simulink model "vx_vy_dekf_v1_12"  (R2024a)
settings: Solver=VariableStepAuto  StartTime=0.0  StopTime=16  RelTol=1e-3
model workspace (MAT data in the model file):
  AVz_bias_v17 = 0
  Ay_bias_v17 = 0
  Q_r_v16 = 0.001
  Q_vy_v16 = 0.0001
  R_Ay_v14 = 0.01
  R_Ay_v15 = 0.01
  R_r_v14 = 0.01
  R_r_v15 = 0.01
  test_speed = 20
  test_steer_amplitude = 0.02
  test_steer_frequency = 0.4
undefined symbols (not defined in the file or in its folder): longitudinal_velocity_estimator_simulink, vy_dekf_v1_12_steer_profile, vy_dynamic_ekf_v1_7
libraries: simulink x4, Solver_SF x1
settings Model: Creator=Xiao Hu  LastModifiedBy=21180

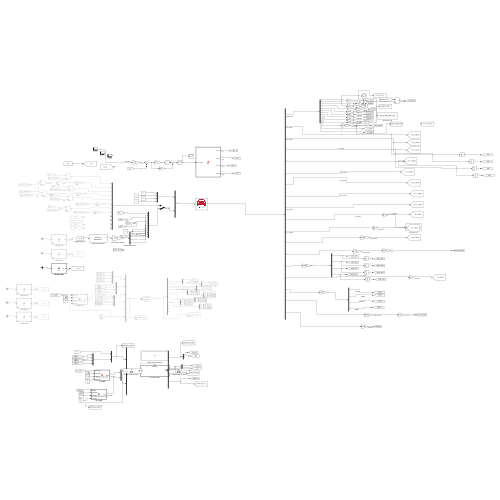
[thumbnail: Simulink's stored preview of the top-level diagram]
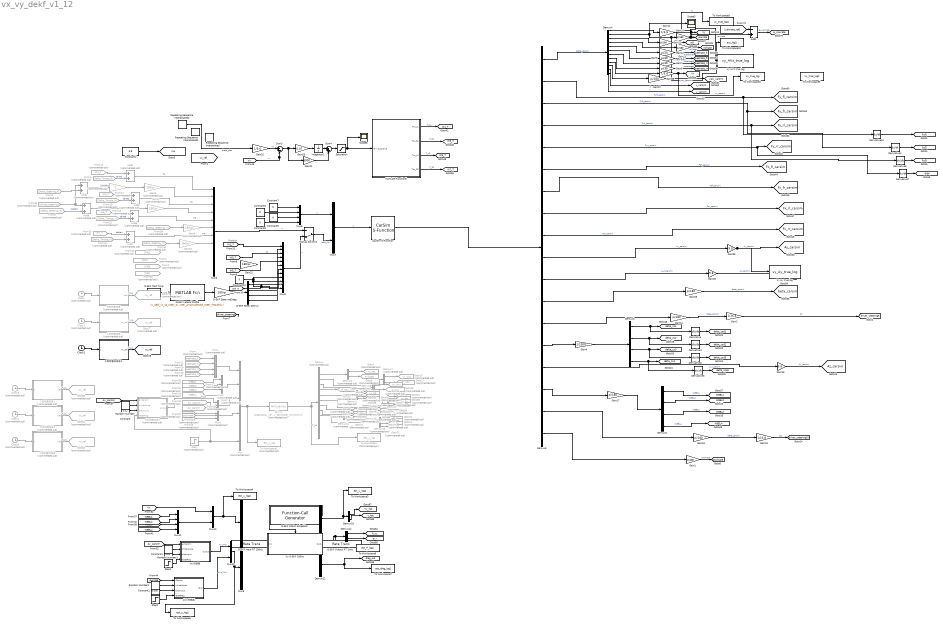
== system vx_vy_dekf_v1_12 ==
  note: Product
  AVz传感器 : MATLAB Function  TreatAsAtomicUnit=on  SystemSampleTime=0.01
  Add1 : Sum  Inputs=-+
  Add{4..9} (6 alike) : Sum  Commented=on
  B高附着加速 : MATLAB Function  Commented=on  TreatAsAtomicUnit=on
  CarSim S-Function : Solver_SF/CarSim S-Function  Priority=1  SIMFILE=simfile.sim  Run_RTs=off  vs_state_ind=Run  StopMode_ind=Vehicle Model
  Clock{,1,3..5} (5 alike) : Clock  Commented=on
  Clock2 : Clock
  Constant : Constant  Value=0.02
  Constant1 : Constant  Value=0.02
  Constant{6..10} (5 alike) : Constant  Value=0
  Constant2 : Constant  Value=0.005
  Constant4 : Constant  Value=0.8
  C高附着减速 : MATLAB Function  Commented=on  TreatAsAtomicUnit=on
  D-EKF 100Hz Scheduler : simulink/Ports & Subsystems/Function-Call Generator  sample_time=0.01  numberOfIterations=1  DisallowWideOutput=off
  D-EKF Input RT 100Hz : RateTransition  OutPortSampleTime=0.01
  D-EKF Lateral Profile : MATLABFcn  MATLABFcn=vy_dekf_v1_12_steer_profile(u,test_steer_amplitude,test_steer_frequency)  OutputDimensions=4  SampleTime=0.001
  D-EKF Output RT 1kHz : RateTransition  OutPortSampleTime=0.001
  D-EKF Steer Demux : Demux
  D-EKF Steer rad2deg : Gain  Gain=180/pi
  D-EKF Test Time : DigitalClock  SampleTime=0.001
  Demux : Demux  Commented=on  Outputs=[2 2 2 1 4 4 4 4 4 2 2 7]
  Demux{1,9..11,13} (5 alike) : Demux  Commented=on
  Demux12 : Demux  Outputs=[2 2 47]
  Demux14 : Demux  Outputs=2
  Demux18 : Demux  Outputs=2
  Demux2 : Demux  Commented=on  Outputs=2
  Demux3 : Demux
  Demux4 : Demux  Outputs=12
  Demux5 : Demux  Outputs=[12 1 1 1 1 1 1 1 1 1 1 1 1 4 1 4 1 1]
  Demux6 : Demux
  Demux7 : Demux  Commented=on  Outputs=2
  Demux8 : Demux  Commented=on  Outputs=2
  Derivative{,1..4,6..7,12} (8 alike) : Derivative
  D高附着加减速1 : MATLAB Function  TreatAsAtomicUnit=on
  From : From  Commented=on  GotoTag=weelrate_fl  TagVisibility=global
  From11 : From  Commented=on  GotoTag=weelrate_fr  TagVisibility=global
  From12 : From  Commented=on  GotoTag=W5_T  TagVisibility=global
  From13 : From  Commented=on  GotoTag=W1_T  TagVisibility=global
  From14 : From  Commented=on  GotoTag=weelrate_rl  TagVisibility=global
  From15 : From  Commented=on  GotoTag=weelrate_rr  TagVisibility=global
  From16 : From  Commented=on  GotoTag=WEEL1  TagVisibility=global
  From17 : From  Commented=on  GotoTag=WEEL3  TagVisibility=global
  From18 : From  Commented=on  GotoTag=WEEL2  TagVisibility=global
  From19 : From  Commented=on  GotoTag=WEEL4  TagVisibility=global
  From2 : From  Commented=on  GotoTag=Fd2  TagVisibility=global
  From20 : From  Commented=on  GotoTag=yawrate  TagVisibility=global
  From21 : From  Commented=on  GotoTag=W3_T  TagVisibility=global
  From22 : From  Commented=on  GotoTag=Delta_Torque_rl  TagVisibility=global
  From23 : From  Commented=on  GotoTag=Delta_Torque_fr  TagVisibility=global
  From24 : From  Commented=on  GotoTag=Delta_Torque_rr  TagVisibility=global
  From25 : From  Commented=on  GotoTag=rollrate  TagVisibility=global
  From26 : From  Commented=on  GotoTag=Ay_carsim  TagVisibility=global
  From28 : From  Commented=on  GotoTag=Az_carsim  TagVisibility=global
  From29 : From  Commented=on  GotoTag=W7_T  TagVisibility=global
  From3 : From  Commented=on  GotoTag=Delta_Torque_fl  TagVisibility=global
  From30 : From  Commented=on  GotoTag=pitchrate  TagVisibility=global
  From35 : From  Commented=on  GotoTag=driver_steering
  From39 : From  Commented=on  GotoTag=Delta_Steering_rl  TagVisibility=global
  From4 : From  Commented=on  GotoTag=Fd3  TagVisibility=global
  From42 : From  Commented=on  GotoTag=Delta_Steering_rr  TagVisibility=global
  From43 : From  Commented=on  GotoTag=Fd1  TagVisibility=global
  From5 : From  Commented=on  GotoTag=Delta_Steering_fl  TagVisibility=global
  From50 : From  Commented=on  GotoTag=Fd4  TagVisibility=global
  From6 : From  Commented=on  GotoTag=Delta_Steering_fr  TagVisibility=global
  F低附着加速1 : MATLAB Function  Commented=on  TreatAsAtomicUnit=on
  F低附着加速2 : MATLAB Function  Commented=on  TreatAsAtomicUnit=on
  Gain{1,10,12,14,17..18,23,29,37} (9 alike) : Gain  Gain=pi/180
  Gain11 : Gain  Gain=1/3.6
  Gain{3,5,9,13} (4 alike) : Gain  Commented=on  Gain=180/pi
  Gain15 : Gain  Gain=1/3.6
  Gain16 : Gain  Gain=9.8
  Gain19 : Gain  Gain=1/16.8
  Gain2 : Gain  Gain=1/16.8
  Gain21 : Gain  Gain=5000
  Gain22 : Gain  Gain=180/pi
  Gain{6..8,24} (4 alike) : Gain  Gain=pi/30
  Gain25 : Gain  Gain=0.07
  Gain28 : Gain  Gain=9.8
  Gain36 : Gain  Gain=9.8
  Gain38 : Gain  Gain=1/3.6
  Gain39 : Gain  Commented=on
  Gain4 : Gain  Gain=1/1000
  Goto10 : Goto  Commented=on  GotoTag=vx_wss  TagVisibility=global
  Goto17 : Goto  Commented=on  GotoTag=P_wss  TagVisibility=global
  Goto28 : Goto  Commented=on  GotoTag=vx_imu  TagVisibility=global
  Goto29 : Goto  Commented=on  GotoTag=P_imu  TagVisibility=global
  Goto30 : Goto  Commented=on  GotoTag=P_wss_imu  TagVisibility=global
  Goto32 : Goto  Commented=on  GotoTag=vx_FL  TagVisibility=global
  Goto38 : Goto  Commented=on  GotoTag=vx_FR  TagVisibility=global
  Goto39 : Goto  Commented=on  GotoTag=vx_RL  TagVisibility=global
  Goto40 : Goto  Commented=on  GotoTag=vx_RR  TagVisibility=global
  Goto41 : Goto  Commented=on  GotoTag=slip_FL  TagVisibility=global
  Goto57 : Goto  Commented=on  GotoTag=slip_FR  TagVisibility=global
  Goto58 : Goto  Commented=on  GotoTag=slip_RL  TagVisibility=global
  Goto59 : Goto  Commented=on  GotoTag=slip_RR  TagVisibility=global
  Goto64 : Goto  Commented=on  GotoTag=rho_FL  TagVisibility=global
  Goto65 : Goto  Commented=on  GotoTag=rho_FR  TagVisibility=global
  Goto66 : Goto  Commented=on  GotoTag=rho_RL  TagVisibility=global
  Goto67 : Goto  Commented=on  GotoTag=rho_RR  TagVisibility=global
  Goto68 : Goto  Commented=on  GotoTag=R_FL  TagVisibility=global
  Goto69 : Goto  Commented=on  GotoTag=R_FR  TagVisibility=global
  Goto7 : Goto  Commented=on  GotoTag=vx_hat  TagVisibility=global
  Goto70 : Goto  Commented=on  GotoTag=R_RL  TagVisibility=global
  Goto71 : Goto  Commented=on  GotoTag=R_RR  TagVisibility=global
  Goto72 : Goto  Commented=on  GotoTag=R_FL  TagVisibility=global
  Goto73 : Goto  Commented=on  GotoTag=R_FR  TagVisibility=global
  Goto74 : Goto  Commented=on  GotoTag=R_RL  TagVisibility=global
  Goto75 : Goto  Commented=on  GotoTag=R_RR  TagVisibility=global
  Goto{76..77,80..82} (5 alike) : Goto  Commented=on  GotoTag=vx_ref  TagVisibility=global
  Goto9 : Goto  Commented=on  GotoTag=P_fused  TagVisibility=global
  G低附着减速2 : MATLAB Function  Commented=on  TreatAsAtomicUnit=on
  H低附着加减速 : MATLAB Function  Commented=on  TreatAsAtomicUnit=on
  Integrator1 : Integrator
  MATLAB Function5 : MATLAB Function  TreatAsAtomicUnit=on
  Manual Switch1 : ManualSwitch  CurrentSetting=0
  Mux : Mux  Commented=on  Inputs=[4 4 3 3 3 1]
  Mux1 : Mux  Commented=on
  Mux10 : Mux  Inputs=[1 4]
  Mux11 : Mux
  Mux12 : Mux  Inputs=2
  Mux2 : Mux  Commented=on
  Mux3 : Mux  Commented=on  Inputs=3
  Mux4 : Mux  Commented=on  Inputs=3
  Mux5 : Mux  Inputs=12
  Mux6 : Mux
  Mux7 : Mux  Inputs=[4,12]
  Mux8 : Mux  Inputs=12
  Mux9 : Mux  Inputs=[5 2]
  Random Number : RandomNumber  Variance=0.000025  Seed=20260819  SampleTime=0.01
  Random Number1 : RandomNumber  Variance=0.000025  Seed=20260819  SampleTime=0.01
  Random Number2 : RandomNumber  Variance=0.000025  Seed=20260819  SampleTime=0.01
  Repeating Sequence Interpolated : simulink/Sources/Repeating Sequence Interpolated  OutValues=[40 40 40 40].'  TimeValues=[0 3 8 16].'  LookUpMeth=Interpolation-Use End Values  tsamp=0.001  OutMin=[]  OutMax=[]  OutDataTypeStr=double  OutputDataTypeScalingMode=double  OutDataType=fixdt(0,8)  OutScaling=2^-10
  Repeating Sequence Interpolated1 : simulink/Sources/Repeating Sequence Interpolated  OutValues=[60 60 60 60].'  TimeValues=[0 3 8 16].'  LookUpMeth=Interpolation-Use End Values  tsamp=0.001  OutMin=[]  OutMax=[]  OutDataTypeStr=double  OutputDataTypeScalingMode=double  OutDataType=fixdt(0,8)  OutScaling=2^-10
  Repeating Sequence Interpolated2 : simulink/Sources/Repeating Sequence Interpolated  OutValues=test_speed*3.6*ones(4,1)  TimeValues=[0 3 8 16].'  LookUpMeth=Interpolation-Use End Values  tsamp=0.001  OutMin=[]  OutMax=[]  OutDataTypeStr=double  OutputDataTypeScalingMode=double  OutDataType=fixdt(0,8)  OutScaling=2^-10
  Saturation : Saturate  UpperLimit=2250  LowerLimit=-2250
  Scope3 : Scope
  Scope8 : Scope
  Step : Step  Commented=on  Time=0.01  Before=1  After=0  SampleTime=0
  Step1 : Step  Time=0.01  Before=1  After=0  SampleTime=0
  Step2 : Step  Time=0.01  Before=1  After=0  SampleTime=0
  Sum3 : Sum  Inputs=|+-
  Sum4 : Sum  Inputs=|++
  To Workspace : ToWorkspace  Commented=on  VariableName=est_y_log  SaveFormat=Timeseries  SampleTime=-1
  To Workspace1 : ToWorkspace  Commented=on  VariableName=est_u_log  SaveFormat=Timeseries  SampleTime=-1
  To Workspace10 : ToWorkspace  VariableName=avz_log1  SaveFormat=Timeseries  SampleTime=-1
  To Workspace2 : ToWorkspace  VariableName=Vx_true_log  SaveFormat=Timeseries  SampleTime=-1
  To Workspace3 : ToWorkspace  VariableName=est_y_log1  SaveFormat=Timeseries  SampleTime=-1
  To Workspace4 : ToWorkspace  VariableName=est_u_log1  SaveFormat=Timeseries  SampleTime=-1
  To Workspace5 : ToWorkspace  VariableName=Vx_true_log2  SaveFormat=Timeseries  SampleTime=-1
  To Workspace6 : ToWorkspace  VariableName=est_z_log1  SaveFormat=Timeseries  SampleTime=-1
  To Workspace7 : ToWorkspace  VariableName=est_diag_log1  SaveFormat=Timeseries  SampleTime=-1
  To Workspace8 : ToWorkspace  VariableName=est_P_log1  SaveFormat=Timeseries  SampleTime=-1
  To Workspace9 : ToWorkspace  VariableName=vy_true_log1  SaveFormat=Timeseries  SampleTime=-1
  Vy AVz true log : ToWorkspace  VariableName=vy_AVz_true_log  SaveFormat=Timeseries  SampleTime=0.01
  Vy Ay true log : ToWorkspace  VariableName=vy_Ay_true_log  SaveFormat=Timeseries  SampleTime=0.01
  Vy D-EKF 100Hz : Subsystem  TreatAsAtomicUnit=on
  ay传感器 : MATLAB Function  TreatAsAtomicUnit=on  SystemSampleTime=0.01
  估计vx : MATLABFcn  Commented=on  MATLABFcn=longitudinal_velocity_estimator_simulink(u)  OutputDimensions=38
  tag scope: Ax_carsim=global, Ay_carsim=global, Az_carsim=global, Fx_fl_carsim=global, Fx_fr_carsim=global, Fx_rl_carsim=global, Fx_rr_carsim=global, Fy_fl_carsim=global, Fy_fr_carsim=global, Fy_rl_carsim=global, Fy_rr_carsim=global, P_r=global, P_vy=global, Vx=global, Vy=global, Vy_hat=global, W1_T=global, W3_T=global, W5_T=global, W7_T=global, WEEL1=global, WEEL2=global, WEEL3=global, WEEL4=global, beta_carsim=global, delta_zs1=global, delta_zs2=global, delta_zs3=global, delta_zs4=global, delta_zsd1=global, delta_zsd2=global, delta_zsd3=global, delta_zsd4=global, diag_out=global, driver_steering10=global, driver_steering5=global, e_yawrate=global, fyd1=global, fyd2=global, fyd3=global, fyd4=global, mu=global, pitchrate=global, r_hat=global, roll=global, rollrate=global, vx_ref=global, weelrate_fl=global, weelrate_fr=global, weelrate_rl=global, weelrate_rr=global, x_carsim=global, y_carsim=global, yaw_carsim=global, yawrate=global
  wires:
  From13/1 -> Add4/1
  Gain14/1 -> Gain2/1  "beta_carsim"
  Add1/1 -> [e_yawrate]  "e_yawrate"
  Gain3/1 -> Mux5/4
  From6/1 -> Add8/2  "delta3"
  [W1_T] -> Mux8/1
  Demux5/7 -> [Fx_fr_carsim]  "Fzfr_carsim"
  Demux3/4 -> Derivative3/1, [delta_zs4]
  From12/1 -> Add6/1
  From35/1 -> Add9/1, Add8/1
  Gain39/1 -> Gain5/1
  Gain13/1 -> Mux5/8
  Demux6/4 -> [WEEL4]  "WEEL4"
  Constant6/1 -> Mux6/2
  Add9/1 -> Gain39/1  "总的转角1"
  Derivative1/1 -> [delta_zsd2]
  Demux5/12 -> Gain29/1
  Demux5/8 -> [Fx_rl_carsim]  "Fzrl_carsim"
  Gain19/1 -> [driver_steering10]  "ds1"
  Add4/1 -> Mux5/1  "T1"
  Gain4/1 -> Demux3/1
  Gain38/1 -> To Workspace2/1, [Vx]  "vx_carsim"
  Gain8/1 -> [weelrate_rr]  "weelrate4"
  Add5/1 -> Mux5/3  "T2"
  Demux6/3 -> [WEEL2]  "WEEL2"
  Mux7/1 -> CarSim S-Function/1  "u"
  Mux8/1 -> Manual Switch1/2  "u"
  From21/1 -> Add5/1
  MATLAB Function5/2(Tor_R1) -> [W3_T]  "T_R1"
  Gain36/1 -> [Ay_carsim], Vy Ay true log/1  "Ay_carsim"
  Derivative3/1 -> [delta_zsd4]
  Gain11/1 -> To Workspace9/1, [Vy]  "Vy"
  Sum4/1 -> Saturation/1
  Gain9/1 -> Mux5/6
  Demux5/4 -> Derivative6/1, [Fy_rl_carsim]  "Fyrl_carsim"
  Gain5/1 -> Mux5/2
  Demux5/16 -> Gain17/1
  Gain21/1 -> Sum4/2
  CarSim S-Function/1 -> Demux5/1
  Derivative4/1 -> [fyd2]
  From39/1 -> Gain9/1
  From22/1 -> Add6/2  "delta3"
  Derivative12/1 -> [fyd1]
  From23/1 -> Add5/2  "delta2"
  Gain18/1 -> Gain19/1  "beta_carsim"
  Gain7/1 -> [weelrate_rl]  "weelrate3"
  Derivative7/1 -> [fyd4]
  Derivative6/1 -> [fyd3]
  Constant9/1 -> Mux6/3
  Mux6/1 -> Mux7/1  "u"
  [W3_T] -> Mux8/3  "q1"
  Gain12/1 -> [roll]  "roll"
  Gain17/1 -> Demux6/1
  Demux5/17 -> Gain18/1
  Demux6/2 -> [WEEL3]  "WEEL3"
  Gain16/1 -> [Az_carsim]  "Ax_carsim"
  Derivative/1 -> [delta_zsd1]
  Demux6/1 -> [WEEL1]  "WEEL1"
  Constant10/1 -> Mux8/12, Mux8/11, Mux8/10, Mux8/9
  MATLAB Function5/4(Tor_R2) -> [W7_T]  "T_R2"
  Demux5/13 -> Gain14/1
  Add6/1 -> Mux5/5  "T3"
  From5/1 -> Add9/2
  From3/1 -> Add4/2  "delta1"
  Demux4/7 -> Gain7/1
  MATLAB Function5/1(Tor_L1) -> [W1_T]  "T_L1"
  Demux3/3 -> Derivative2/1, [delta_zs3]
  Demux5/6 -> [Fx_fl_carsim]  "Fzfl_carsim"
  Constant4/1 -> [mu]
  Integrator1/1 -> Sum4/1
  Demux4/3 -> Gain12/1
  Demux5/5 -> [Fy_rr_carsim], Derivative7/1  "Fyrr_carsim"
  Demux4/6 -> Gain6/1
  Derivative2/1 -> [delta_zsd3]
  Gain2/1 -> [driver_steering5]  "ds"
  Demux4/11 -> [x_carsim]  "X"
  Constant8/1 -> Mux6/4
  Demux5/2 -> Derivative12/1, [Fy_fl_carsim]  "Fyfl_carsim"
  Gain6/1 -> [weelrate_fr]  "weelrate2"
  Demux5/1 -> Demux4/1  "delta_carsim"
  Demux5/11 -> Gain28/1  "w_rl_carsim"
  Demux4/5 -> Gain24/1
  Demux5/14 -> Gain4/1
  Add7/1 -> Mux5/7  "T4"
  Manual Switch1/1 -> Mux7/2  "add_Mz"
  Demux5/3 -> Derivative4/1, [Fy_fr_carsim]  "Fyfr_carsim"
  From24/1 -> Add7/2
  Demux4/12 -> [y_carsim]  "Y"
  Demux4/4 -> Gain23/1
  Demux4/2 -> Scope3/1, To Workspace10/1, Gain10/1
  Demux4/8 -> Gain8/1
  Demux5/10 -> Gain36/1  "Ay_carsim"
  Gain25/1 -> Integrator1/1
  Demux3/2 -> Derivative1/1, [delta_zs2]
  From29/1 -> Add7/1  "delta4"
  Gain37/1 -> [yaw_carsim]  "yaw_carsim"
  [driver_steering] -> ?
  Demux4/9 -> Gain38/1
  Demux3/1 -> Derivative/1, [delta_zs1]
  [W7_T] -> Mux8/7  "q1"
  [Vx] -> Sum3/2  "vx"
  Demux5/15 -> Gain16/1  "w_rl_carsim"
  Demux4/1 -> Gain11/1
  Gain28/1 -> [Ax_carsim]  "Ax_carsim"
  Gain24/1 -> [weelrate_fl]  "轮速实际值"
  From42/1 -> Gain13/1
  Constant7/1 -> Mux6/1
  Gain10/1 -> Add1/2, [yawrate], Vy AVz true log/1  "yawrate"
  [W5_T] -> Mux8/5
  Gain29/1 -> [beta_carsim]  "beta_carsim"
  Sum3/1 -> Gain25/1, Gain21/1
  Gain23/1 -> [rollrate]  "rollrate"
  MATLAB Function5/3(Tor_L2) -> [W5_T]  "T_L2"
  Mux5/1 -> Manual Switch1/1  "u"
  Add8/1 -> Gain3/1  "总的转角2"
  Demux4/10 -> Gain37/1
  Demux5/9 -> [Fx_rr_carsim]  "Fzrr_carsim"
  [yawrate_ref] -> Add1/1
  Mux/1 -> 估计vx/1, To Workspace1/1
  Mux1/1 -> Mux/1
  From/1 -> Mux1/1
  From11/1 -> Mux1/2
  From14/1 -> Mux1/3
  From15/1 -> Mux1/4
  From16/1 -> Mux2/1
  From17/1 -> Mux2/2
  From18/1 -> Mux2/3
  From19/1 -> Mux2/4
  Mux2/1 -> Mux/2
  Mux3/1 -> Mux/3
  Mux4/1 -> Mux/4
  Gain1/1 -> [pitchrate]  "pitchrate"
  Demux5/18 -> Gain1/1
  [Ax_carsim] -> F低附着加速2/1(axCarsim)
  From26/1 -> Mux3/2
  From28/1 -> Mux3/3
  From20/1 -> Mux4/1
  From30/1 -> Mux4/2
  From25/1 -> Mux4/3
  估计vx/1 -> Demux/1, To Workspace/1  "T_L1"
  Demux/1 -> Demux2/1
  Demux2/1 -> Goto7/1
  Demux2/2 -> Goto9/1
  Demux7/1 -> Goto10/1
  Demux/2 -> Demux7/1
  Demux7/2 -> Goto17/1
  Demux/3 -> Demux8/1
  Demux8/2 -> Goto29/1
  Demux8/1 -> Goto28/1
  Demux/4 -> Goto30/1
  Demux1/1 -> Goto32/1
  Demux1/2 -> Goto38/1
  Demux1/3 -> Goto39/1
  Demux1/4 -> Goto40/1
  Demux/5 -> Demux1/1
  Demux9/3 -> Goto58/1
  Demux/6 -> Demux9/1
  Demux9/4 -> Goto59/1
  Demux9/2 -> Goto57/1
  Demux9/1 -> Goto41/1
  Demux/7 -> Demux10/1
  Demux10/3 -> Goto66/1
  Demux10/1 -> Goto64/1
  Demux10/4 -> Goto67/1
  Demux10/2 -> Goto65/1
  Demux11/3 -> Goto70/1
  Demux11/4 -> Goto71/1
  Demux/8 -> Demux11/1
  Demux11/2 -> Goto69/1
  Demux11/1 -> Goto68/1
  Demux13/2 -> Goto73/1
  Demux/9 -> Demux13/1
  Demux13/3 -> Goto74/1
  Demux13/4 -> Goto75/1
  Demux13/1 -> Goto72/1
  Step/1 -> F低附着加速2/4(resetFlag), Mux/6
  Repeating Sequence Interpolated2/1 -> Gain15/1  "theta_des"
  Gain15/1 -> Sum3/1  "Vy"
  Clock/1 -> B高附着加速/1(t)
  B高附着加速/1(vref) -> Goto76/1  "T_L1"
  C高附着减速/1(Vx_ref) -> Goto77/1  "T_L1"
  Clock1/1 -> C高附着减速/1(t)
  Clock2/1 -> D高附着加减速1/1(t)
  D高附着加减速1/1(Vx_ref) -> [vx_ref]  "T_L1"
  Clock3/1 -> F低附着加速1/1(t)
  F低附着加速1/1(vref) -> Goto80/1  "T_L1"
  Saturation/1 -> Scope8/1, MATLAB Function5/1(Drive_torque)
  G低附着减速2/1(vref) -> Goto81/1  "T_L1"
  Clock4/1 -> G低附着减速2/1(t)
  H低附着加减速/1(vref) -> Goto82/1  "T_L1"
  Clock5/1 -> H低附着加减速/1(t)
  Constant/1 -> F低附着加速2/3(biasInput)
  Random Number/1 -> F低附着加速2/2(whiteNoise)
  F低附着加速2/1(axOut) -> Mux3/1  "T_L1"
  [Ay_carsim] -> ay传感器/1(ayCarsim)
  Demux18/2 -> [r_hat]
  Demux12/3 -> [diag_out], To Workspace7/1
  Demux12/1 -> To Workspace3/1, Demux18/1
  Step1/1 -> ay传感器/4(resetFlag)
  Constant1/1 -> ay传感器/3(biasInput)
  [WEEL3] -> Mux11/3
  [WEEL4] -> Mux11/4
  Random Number1/1 -> ay传感器/2(whiteNoise)
  [WEEL2] -> Mux11/2
  [WEEL1] -> Mux11/1
  Mux11/1 -> Mux10/2
  [Vx] -> Mux10/1
  Mux10/1 -> To Workspace4/1, Mux9/1
  ay传感器/1(ayOut) -> Mux12/1  "Ay_IMU"
  Mux12/1 -> Mux9/2, To Workspace6/1
  Random Number2/1 -> AVz传感器/2(whiteNoise)
  Constant2/1 -> AVz传感器/3(biasInput)
  Step2/1 -> AVz传感器/4(resetFlag)
  [yawrate] -> AVz传感器/1(rCarsim)
  AVz传感器/1(rOut) -> Mux12/2  "AVz_IMU"
  Demux18/1 -> [Vy_hat]
  Demux14/2 -> [P_r]
  Demux14/1 -> [P_vy]
  Demux12/2 -> To Workspace8/1, Demux14/1
  Mux9/1 -> D-EKF Input RT 100Hz/1
  D-EKF Input RT 100Hz/1 -> Vy D-EKF 100Hz/1(In1)
  D-EKF 100Hz Scheduler/1 -> Vy D-EKF 100Hz/Trigger
  Vy D-EKF 100Hz/1(Out1) -> D-EKF Output RT 1kHz/1
  D-EKF Output RT 1kHz/1 -> Demux12/1
  D-EKF Test Time/1 -> D-EKF Lateral Profile/1
  D-EKF Lateral Profile/1 -> D-EKF Steer rad2deg/1
  D-EKF Steer rad2deg/1 -> D-EKF Steer Demux/1
  D-EKF Steer Demux/1 -> Mux8/2
  D-EKF Steer Demux/2 -> Mux8/4
  D-EKF Steer Demux/3 -> Mux8/6
  D-EKF Steer Demux/4 -> Mux8/8

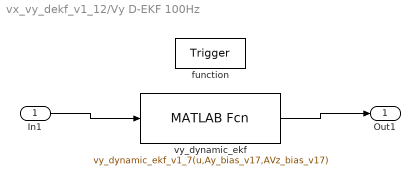
== system vx_vy_dekf_v1_12/Vy D-EKF 100Hz ==
  In1 : Inport
  function : TriggerPort  TriggerType=function-call  VariantControl=(inherit)
  vy_dynamic_ekf : MATLABFcn  MATLABFcn=vy_dynamic_ekf_v1_7(u,Ay_bias_v17,AVz_bias_v17)  OutputDimensions=51
  Out1 : Outport
  wires:
  In1/1 -> vy_dynamic_ekf/1
  vy_dynamic_ekf/1 -> Out1/1

== matlab function vx_vy_dekf_v1_12/B高附着加速 ==
  data: vref output; t input
function vref = fcn(t)

v0 = 60;
v1 = 100;

t1 = 3;
t2 = 8;

if t <= t1

    vref = v0;

elseif t < t2

    tau = (t-t1)/(t2-t1);

    s = 10*tau^3 ...
      - 15*tau^4 ...
      + 6*tau^5;

    vref = v0 + ...
        (v1-v0)*s;

else

    vref = v1;

end

== matlab function vx_vy_dekf_v1_12/C高附着减速 ==
  data: Vx_ref output; t input
function Vx_ref = fcn(t)
%#codegen
% 工况C：高附着直线平滑减速
% 0~3 s   : 100 km/h
% 3~8 s   : 100 -> 60 km/h
% 8~15 s  : 60 km/h
%
% 输出 Vx_ref 单位：m/s

v0 = 100;      % 27.7778 m/s
v1 = 60 ;       % 16.6667 m/s

t1 = 3.0;
t2 = 8.0;

if t <= t1

    Vx_ref = v0;

elseif t < t2

    tau = (t - t1) / (t2 - t1);

    s = 10*tau^3 - 15*tau^4 + 6*tau^5;

    Vx_ref = v0 + (v1 - v0)*s;

else

    Vx_ref = v1;

end
end

== matlab function vx_vy_dekf_v1_12/D高附着加减速1 ==
  data: Vx_ref output; t input
function Vx_ref = fcn(t)
%#codegen
% 加速-减速组合工况
%
% 0~3 s    : 60 km/h 匀速
% 3~8 s    : 60 -> 100 km/h 平滑加速
% 8~13 s   : 100 -> 60 km/h 平滑减速
% 13~16 s  : 60 km/h 匀速
%
% 输出 Vx_ref 单位：m/s

v_low  = 60;      % 16.6667 m/s
v_high = 100;
t1 = 3.0;
t2 = 8.0;
t3 = 13.0;

if t <= t1

    % 0~3 s：60 km/h 匀速
    Vx_ref = v_low;

elseif t < t2

    % 3~8 s：60 -> 100 km/h
    tau = (t - t1) / (t2 - t1);

    s = 10*tau^3 ...
      - 15*tau^4 ...
      + 6*tau^5;

    Vx_ref = v_low + (v_high - v_low)*s;

elseif t < t3

    % 8~13 s：100 -> 60 km/h
    tau = (t - t2) / (t3 - t2);

    s = 10*tau^3 ...
      - 15*tau^4 ...
      + 6*tau^5;

    Vx_ref = v_high + (v_low - v_high)*s;

else

    % 13~16 s：60 km/h 匀速
    Vx_ref = v_low;

end

end

== matlab function vx_vy_dekf_v1_12/F低附着加速1 ==
  data: vref output; t input
function vref = fcn(t)

% mu = 0.3
% 0~3 s : 40 km/h
% 3~8 s : 40 -> 70 km/h
% 8s以后: 70 km/h

v0 = 40;
v1 = 70;

t1 = 3;
t2 = 8;

if t <= t1

    vref_kmh = v0;

elseif t < t2

    tau = (t-t1)/(t2-t1);

    s = 10*tau^3 ...
      - 15*tau^4 ...
      + 6*tau^5;

    vref_kmh = v0 + ...
        (v1-v0)*s;

else

    vref_kmh = v1;

end

vref = vref_kmh;

end

== matlab function vx_vy_dekf_v1_12/G低附着减速2 ==
  data: vref output; t input
function vref = fcn(t)

% mu = 0.3
% 低附着平滑减速工况
%
% 0~3 s : 70 km/h
% 3~8 s : 70 -> 40 km/h
% 8s以后: 40 km/h
%
% 输出单位：km/h

v0 = 70;
v1 = 40;

t1 = 3;
t2 = 8;

if t <= t1

    vref_kmh = v0;

elseif t < t2

    tau = (t-t1)/(t2-t1);

    s = 10*tau^3 ...
      - 15*tau^4 ...
      + 6*tau^5;

    vref_kmh = v0 + ...
        (v1-v0)*s;

else

    vref_kmh = v1;

end

vref = vref_kmh;

end

== matlab function vx_vy_dekf_v1_12/H低附着加减速 ==
  data: vref output; t input
function vref = fcn(t)

% mu = 0.3
% 低附着加速-减速组合工况
%
% 0~3 s    : 40 km/h
% 3~8 s    : 40 -> 70 km/h
% 8~13 s   : 70 -> 40 km/h
% 13~16 s  : 40 km/h
%
% 输出单位：km/h

v_low  = 40;
v_high = 70;

t1 = 3;
t2 = 8;
t3 = 13;

if t <= t1

    % 0~3 s：40 km/h 匀速
    vref_kmh = v_low;

elseif t < t2

    % 3~8 s：40 -> 70 km/h 平滑加速
    tau = (t-t1)/(t2-t1);

    s = 10*tau^3 ...
      - 15*tau^4 ...
      + 6*tau^5;

    vref_kmh = v_low + ...
        (v_high-v_low)*s;

elseif t < t3

    % 8~13 s：70 -> 40 km/h 平滑减速
    tau = (t-t2)/(t3-t2);

    s = 10*tau^3 ...
      - 15*tau^4 ...
      + 6*tau^5;

    vref_kmh = v_high + ...
        (v_low-v_high)*s;

else

    % 13~16 s：40 km/h 匀速
    vref_kmh = v_low;

end

vref = vref_kmh;

end

== matlab function vx_vy_dekf_v1_12/F低附着加速2 ==
  data: axOut output; axCarsim input; whiteNoise input; biasInput input; resetFlag input
function axOut = imu_ax_preprocess( ...
    axCarsim, whiteNoise, biasInput, resetFlag)
%#codegen
%
% IMU纵向加速度传感器模型 + 因果低通预处理
%
% 输入：
%   axCarsim   : CarSim理想纵向加速度 [m/s^2]
%   whiteNoise : Random Number生成的白噪声 [m/s^2]
%   biasInput  : IMU残余bias [m/s^2]
%   resetFlag  : 与估计器reset一致
%
% 输出：
%   axOut      : 最终送入est_u(9)的IMU Ax
%
% 本模块按100Hz设计。

persistent yPrev

%% =========================================================
% 参数
% ==========================================================

Ts = 0.01;

% 第一版20 Hz低通
fc = 20.0;

%% =========================================================
% 输入数值保护
% ==========================================================

if ~isfinite(axCarsim)
    axCarsim = 0;
end

if ~isfinite(whiteNoise)
    whiteNoise = 0;
end

if ~isfinite(biasInput)
    biasInput = 0;
end

%% =========================================================
% 构造非理想IMU测量
%
% a_meas = a_true + bias + noise
% ==========================================================

axMeasured = ...
    axCarsim + ...
    biasInput + ...
    whiteNoise;

%% =========================================================
% 一阶因果低通参数
% ==========================================================

tau = ...
    1/(2*pi*fc);

alpha = ...
    Ts/(tau+Ts);

%% =========================================================
% 初始化 / reset
% ==========================================================

if isempty(yPrev)

    yPrev = axMeasured;

end

if resetFlag > 0.5

    yPrev = axMeasured;

end

%% =========================================================
% 因果一阶低通
%
% y[k] = y[k-1] + alpha*(x[k]-y[k-1])
% ==========================================================

axOut = ...
    yPrev + ...
    alpha*(axMeasured-yPrev);

%% =========================================================
% 保存
% ==========================================================

yPrev = axOut;

end

== matlab function vx_vy_dekf_v1_12/AVz传感器 ==
  data: rOut output; rCarsim input; whiteNoise input; biasInput input; resetFlag input
function rOut = imu_yawrate_preprocess( ...
    rCarsim, whiteNoise, biasInput, resetFlag)
%#codegen
%
% IMU横摆角速度传感器模型 + 一阶因果低通
%
% 输入：
%   rCarsim    : CarSim理想横摆角速度 AVz [rad/s]
%   whiteNoise : 陀螺仪白噪声 [rad/s]
%   biasInput  : 陀螺仪bias [rad/s]
%   resetFlag  : reset信号
%
% 输出：
%   rOut       : IMU处理后的横摆角速度 [rad/s]
%
% Sample time:
%   Ts = 0.01s
%   100Hz
%

persistent yPrev


%% ================================
% 参数
% ================================

Ts = 0.01;


% 陀螺仪低通截止频率
fc = 20;


%% ================================
% 初始化
% ================================

if isempty(yPrev)

    yPrev = 0;

end


%% ================================
% 数值保护
% ================================

if ~isfinite(rCarsim)

    rCarsim = 0;

end


if ~isfinite(whiteNoise)

    whiteNoise = 0;

end


if ~isfinite(biasInput)

    biasInput = 0;

end


if ~isfinite(resetFlag)

    resetFlag = 0;

end


%% ================================
% 构造IMU测量
%
% r_meas = r_true + bias + noise
%
% ================================

rMeasured = ...
    rCarsim + ...
    biasInput + ...
    whiteNoise;



%% ================================
% 一阶低通
%
% alpha = Ts/(tau+Ts)
%
% ================================

tau = ...
    1/(2*pi*fc);


alpha = ...
    Ts/(tau+Ts);



%% ================================
% reset
% ================================

if resetFlag > 0.5

    rOut = rMeasured;

else

    rOut = yPrev + ...
        alpha*(rMeasured-yPrev);

end



%% ================================
% 保存状态
% ================================

yPrev = rOut;


end

== matlab function vx_vy_dekf_v1_12/ay传感器 ==
  data: ayOut output; ayCarsim input; whiteNoise input; biasInput input; resetFlag input
function ayOut = imu_ay_preprocess( ...
    ayCarsim, whiteNoise, biasInput, resetFlag)
%#codegen
%
% IMU纵向加速度传感器模型 + 因果低通预处理
%
% 输入：
%   axCarsim   : CarSim理想纵向加速度 [m/s^2]
%   whiteNoise : Random Number生成的白噪声 [m/s^2]
%   biasInput  : IMU残余bias [m/s^2]
%   resetFlag  : 与估计器reset一致
%
% 输出：
%   axOut      : 最终送入est_u(9)的IMU Ax
%
% 本模块按100Hz设计。

persistent yPrev

%% =========================================================
% 参数
% ==========================================================

Ts = 0.01;

% 第一版20 Hz低通
fc = 20.0;

%% =========================================================
% 输入数值保护
% ==========================================================

if ~isfinite(ayCarsim)
    ayCarsim = 0;
end

if ~isfinite(whiteNoise)
    whiteNoise = 0;
end

if ~isfinite(biasInput)
    biasInput = 0;
end

%% =========================================================
% 构造非理想IMU测量
%
% a_meas = a_true + bias + noise
% ==========================================================

axMeasured = ...
    ayCarsim + ...
    biasInput + ...
    whiteNoise;

%% =========================================================
% 一阶因果低通参数
% ==========================================================

tau = ...
    1/(2*pi*fc);

alpha = ...
    Ts/(tau+Ts);

%% =========================================================
% 初始化 / reset
% ==========================================================

if isempty(yPrev)

    yPrev = axMeasured;

end

if resetFlag > 0.5

    yPrev = axMeasured;

end

%% =========================================================
% 因果一阶低通
%
% y[k] = y[k-1] + alpha*(x[k]-y[k-1])
% ==========================================================

ayOut = ...
    yPrev + ...
    alpha*(axMeasured-yPrev);

%% =========================================================
% 保存
% ==========================================================

yPrev = ayOut;

end

== matlab function vx_vy_dekf_v1_12/MATLAB Function5 ==
  data: Tor_L1 output; Tor_R1 output; Tor_L2 output; Tor_R2 output; Drive_torque input
function [Tor_L1,Tor_R1,Tor_L2,Tor_R2] = fcn(Drive_torque)

%L2左轮到右轮宽度
%deltaMxL1,deltaMxL2,deltaMxR1,deltaMxR2:分别是前左，后左，前右，后右的附加横摆力矩增量。和驱动力使用的驱动力矩相加就是总的轮胎力
%Rwheel,轮胎滚动半径


Tor_L1 = 0.25*Drive_torque;
Tor_L2 = 0.25*Drive_torque;
Tor_R1 = 0.25*Drive_torque;
Tor_R2 = 0.25*Drive_torque;
